simulink subsystem "TV_FLC"  (R2026a)
settings: Solver=VariableStepAuto
model mask{StrWheelRatio=Control.StrWheelRatio, Ku=Control.UndersteerGradient, L=Control.Wheelbase, rwheel=Control.WheelRad, Gr=Control.GearRatio, fis=Control.FuzzySystem, Kp=Control.KpMoment, tr=Control.RearTrack, alpha_max=Control.SlipTh, MotorT=Control.MotorTrq, MotorW=Control.MotorW, F=Control.F, Tmax=max(Control.MotorTrq)}
  mask prompts: StrWheelRatio "Steering Ratio"; Ku "Understeer Gradient"; L "WheelBase"; rwheel "Wheel Radius"; Gr "Gear ratio"; fis "Fuzzy Inference System"; Kp "Moment Coef"; tr "Rear Track"; alpha_max "Slip Threshold"; MotorT "Motor Map Torque"; MotorW "Motor Map RPM"; F "Moment to torque"; Tmax "Max Torque"
values from neighbouring files (symbols this model uses):
  Gr = 1/Vehicle.Powertrain.Driveline.Gearbox.ratio.Value    [sm_car_controlparam_FLCDYC.m]
  L = -Vehicle.Chassis.Body.sAxle2.Value(1)    [sm_car_controlparam_FLCDYC.m]
  rwheel = tire_param.DIMENSION.UNLOADED_RADIUS    [sm_car_controlparam_FLCDYC.m]
  tr = Vehicle.Chassis.Body.TrackRear.Value    [sm_car_controlparam_FLCDYC.m]
libraries: sl_discontinuities x7, simulink x1, fuzblock x1
settings Model: Creator=andrei  LastModifiedBy=andrei

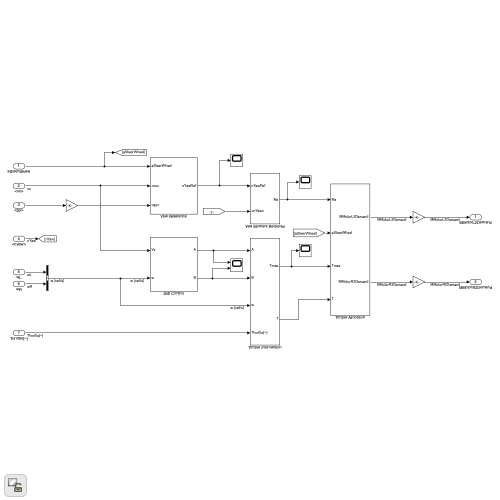
[thumbnail: Simulink's stored preview of the top-level diagram]
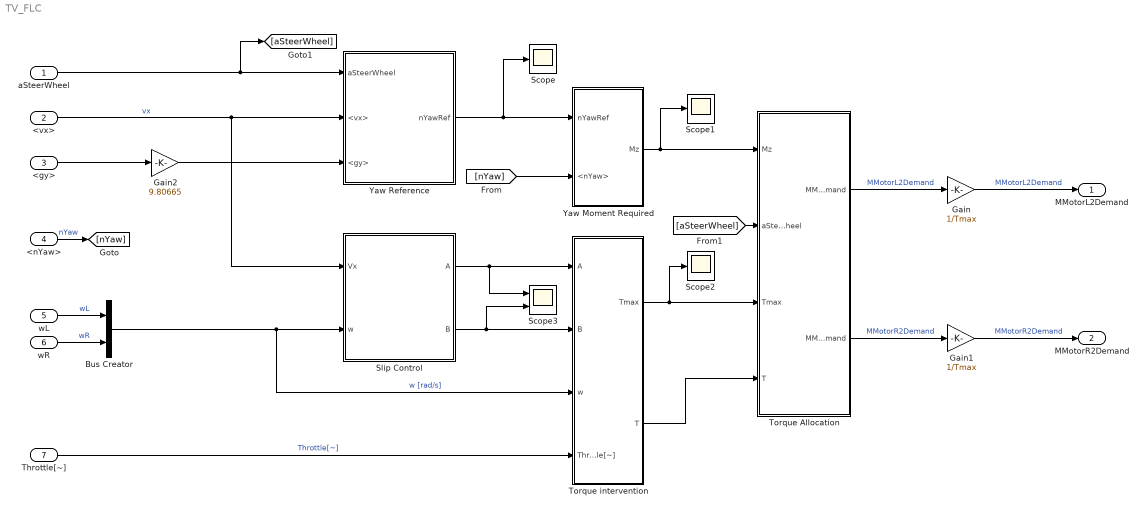
== system TV_FLC ==
  aSteerWheel : Inport  OutDataTypeStr=double  PortDimensions=1  SampleTime=0
  <vx> : Inport  Port=2  OutDataTypeStr=double  PortDimensions=1  SampleTime=0
  <gy> : Inport  Port=3  OutDataTypeStr=double  PortDimensions=1  SampleTime=0
  <nYaw> : Inport  Port=4  OutDataTypeStr=double  PortDimensions=1  SampleTime=0
  wL : Inport  Port=5  OutDataTypeStr=double  PortDimensions=1  SampleTime=0
  wR : Inport  Port=6  OutDataTypeStr=double  PortDimensions=1  SampleTime=0
  Throttle[~] : Inport  Port=7  OutDataTypeStr=double  PortDimensions=1  SampleTime=0
  Bus Creator : BusCreator  Inputs=2
  Gain : Gain  Gain=1/Tmax
  Gain1 : Gain  Gain=1/Tmax
  Gain2 : Gain  Gain=9.80665
  Scope : Scope
      settings: ActiveDisplayYMinimum=-0.70950113712266094  ActiveDisplayYMaximum=0.73291856494418972  DataLoggingVariableName=ScopeData12
  Scope1 : Scope
      settings: ActiveDisplayYMinimum=-1  ActiveDisplayYMaximum=1  DataLoggingVariableName=ScopeData13
  Scope2 : Scope
      settings: ActiveDisplayYMinimum=-1  ActiveDisplayYMaximum=1  DataLoggingVariableName=ScopeData3
  Scope3 : Scope  NumInputPorts=2
      settings: ActiveDisplayYMinimum=-0.025466589931511983  ActiveDisplayYMaximum=0.22919930938361235  DataLoggingVariableName=ScopeData9
  Slip Control : Subsystem
  Torque Allocation : Subsystem
  Torque intervention : Subsystem
  Yaw Moment Required : Subsystem
  Yaw Reference : Subsystem
  MMotorL2Demand : Outport  OutDataTypeStr=double  PortDimensions=1  SampleTime=0
  MMotorR2Demand : Outport  Port=2  OutDataTypeStr=double  PortDimensions=1  SampleTime=0
  wires:
  Torque Allocation/1(MMotorL2Demand) -> Gain/1  "MMotorL2Demand"
  <vx>/1 -> Yaw Reference/2(<vx>), Slip Control/1(Vx)  "vx"
  Slip Control/2(B) -> Torque intervention/2(B), Scope3/2
  <nYaw>/1 -> [nYaw]  "nYaw"
  Slip Control/1(A) -> Torque intervention/1(A), Scope3/1
  wL/1 -> Bus Creator/1  "wL"
  Yaw Moment Required/1(Mz) -> Torque Allocation/1(Mz), Scope1/1
  Throttle[~]/1 -> Torque intervention/4(Throttle[~])  "Throttle[~]"
  <gy>/1 -> Gain2/1
  Gain1/1 -> MMotorR2Demand/1  "MMotorR2Demand"
  [nYaw] -> Yaw Moment Required/2(<nYaw>)
  Bus Creator/1 -> Slip Control/2(w), Torque intervention/3(w)  "w [rad/s]"
  Gain/1 -> MMotorL2Demand/1  "MMotorL2Demand"
  Torque Allocation/2(MMotorR2Demand) -> Gain1/1  "MMotorR2Demand"
  Yaw Reference/1(nYawRef) -> Yaw Moment Required/1(nYawRef), Scope/1
  wR/1 -> Bus Creator/2  "wR"
  Torque intervention/1(Tmax) -> Torque Allocation/3(Tmax), Scope2/1
  Gain2/1 -> Yaw Reference/3(<gy>)
  Torque intervention/2(T) -> Torque Allocation/4(T)
  aSteerWheel/1 -> [aSteerWheel], Yaw Reference/1(aSteerWheel)
  [aSteerWheel] -> Torque Allocation/2(aSteerWheel)

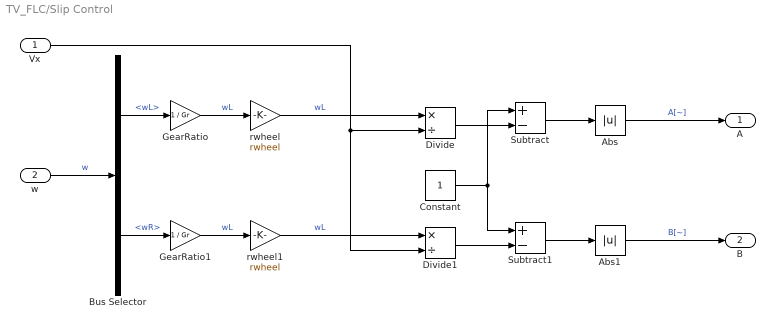
== system TV_FLC/Slip Control ==
  Vx : Inport
  w : Inport  Port=2
  Abs : Abs  SaturateOnIntegerOverflow=off
  Abs1 : Abs  SaturateOnIntegerOverflow=off
  Bus Selector : BusSelector  OutputSignals=wL,wR
  Constant : Constant
  Divide : Product  Inputs=*/
  Divide1 : Product  Inputs=*/
  GearRatio : Gain  Gain=1 / Gr
  GearRatio1 : Gain  Gain=1 / Gr
  Subtract : Sum  Inputs=+-
  Subtract1 : Sum  Inputs=+-
  rwheel : Gain  Gain=rwheel
  rwheel1 : Gain  Gain=rwheel
  A : Outport
  B : Outport  Port=2
  wires:
  GearRatio1/1 -> rwheel1/1  "wL"
  GearRatio/1 -> rwheel/1  "wL"
  rwheel1/1 -> Divide1/1  "wL"
  Bus Selector/1 -> GearRatio/1  "<wL>"
  w/1 -> Bus Selector/1  "w"
  Vx/1 -> Divide1/2, Divide/2
  Subtract/1 -> Abs/1
  Subtract1/1 -> Abs1/1
  rwheel/1 -> Divide/1  "wL"
  Bus Selector/2 -> GearRatio1/1  "<wR>"
  Constant/1 -> Subtract/1, Subtract1/1
  Divide/1 -> Subtract/2
  Divide1/1 -> Subtract1/2
  Abs/1 -> A/1  "A[~]"
  Abs1/1 -> B/1  "B[~]"

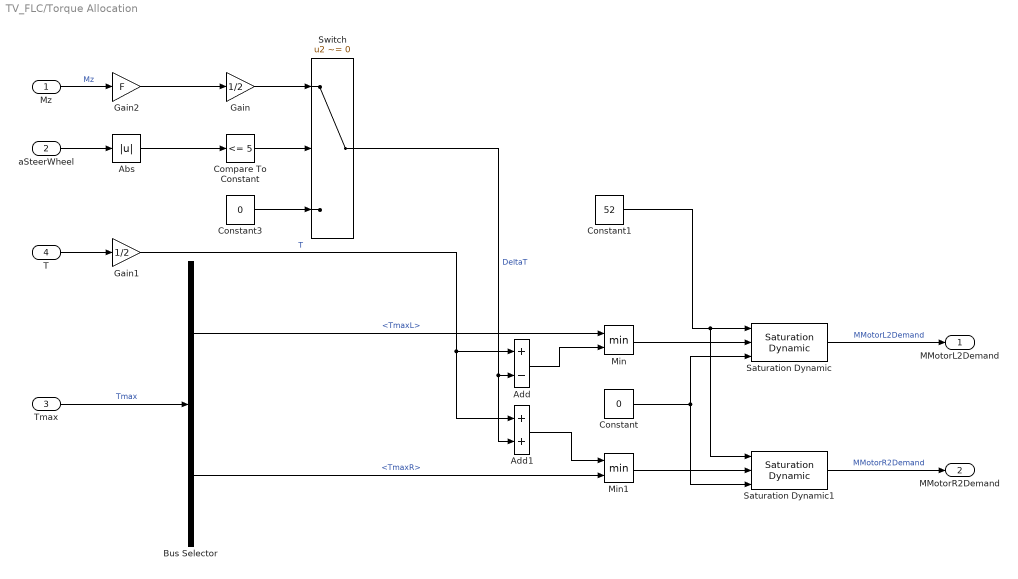
== system TV_FLC/Torque Allocation ==
  Mz : Inport
  aSteerWheel : Inport  Port=2
  Tmax : Inport  Port=3
  T : Inport  Port=4
  Abs : Abs  SaturateOnIntegerOverflow=off
  Add : Sum  Inputs=+-
  Add1 : Sum
  Bus Selector : BusSelector  OutputSignals=TmaxL,TmaxR
  Compare To Constant : simulink/Logic and Bit Operations/Compare To Constant  relop=<=  const=5  OutDataTypeStr=boolean
  Constant : Constant  Value=0
  Constant1 : Constant  Value=52
  Constant3 : Constant  Value=0
  Gain : Gain  Gain=1/2
  Gain1 : Gain  Gain=1/2
  Gain2 : Gain  Gain=F
  Min : MinMax  Inputs=2
  Min1 : MinMax  Inputs=2
  Saturation Dynamic : sl_discontinuities/Saturation Dynamic  OutMin=[]  OutMax=[]  OutDataTypeStr=Inherit: Same as second input  OutDataType=fixdt(1, 16)  OutScaling=2^-10  DoSatur=off
  Saturation Dynamic1 : sl_discontinuities/Saturation Dynamic  OutMin=[]  OutMax=[]  OutDataTypeStr=Inherit: Same as second input  OutDataType=fixdt(1, 16)  OutScaling=2^-10  DoSatur=off
  Switch : Switch  Criteria=u2 ~= 0  SaturateOnIntegerOverflow=off  InputSameDT=off
  MMotorL2Demand : Outport
  MMotorR2Demand : Outport  Port=2
  wires:
  Constant1/1 -> Saturation Dynamic/1, Saturation Dynamic1/1
  Gain2/1 -> Gain/1
  Min/1 -> Saturation Dynamic/2
  Min1/1 -> Saturation Dynamic1/2
  Gain/1 -> Switch/1
  Compare To Constant/1 -> Switch/2
  aSteerWheel/1 -> Abs/1
  Switch/1 -> Add/2, Add1/2  "DeltaT"
  Abs/1 -> Compare To Constant/1
  Constant3/1 -> Switch/3
  Constant/1 -> Saturation Dynamic1/3, Saturation Dynamic/3
  T/1 -> Gain1/1
  Mz/1 -> Gain2/1  "Mz"
  Gain1/1 -> Add/1, Add1/1  "T"
  Add1/1 -> Min1/1
  Add/1 -> Min/2
  Saturation Dynamic/1 -> MMotorL2Demand/1  "MMotorL2Demand"
  Saturation Dynamic1/1 -> MMotorR2Demand/1  "MMotorR2Demand"
  Tmax/1 -> Bus Selector/1  "Tmax"
  Bus Selector/1 -> Min/1  "<TmaxL>"
  Bus Selector/2 -> Min1/2  "<TmaxR>"

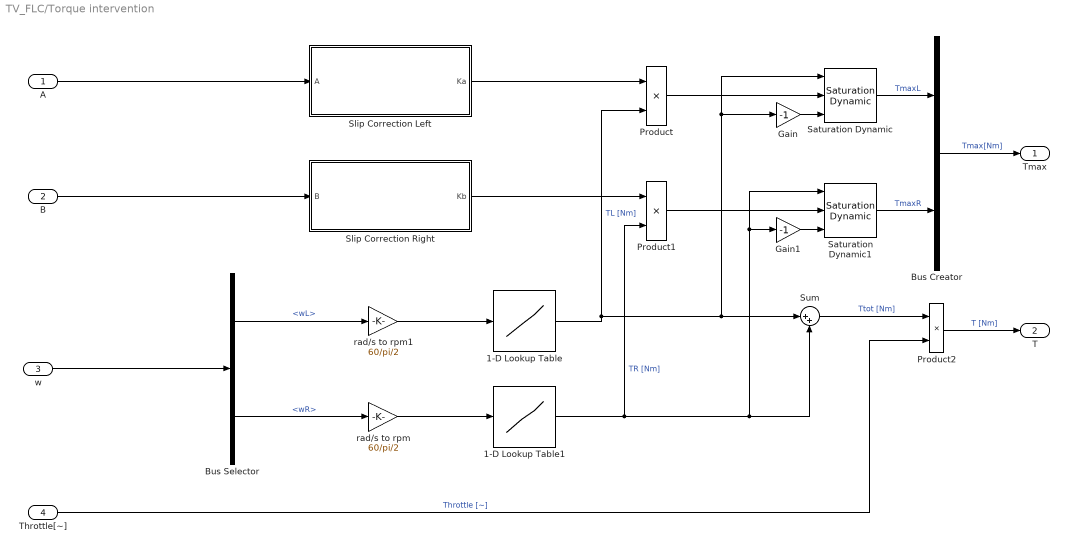
== system TV_FLC/Torque intervention ==
  A : Inport
  B : Inport  Port=2
  w : Inport  Port=3
  Throttle[~] : Inport  Port=4
  1-D Lookup Table : Lookup_n-D  NumberOfTableDimensions=1  BreakpointsForDimension1=MotorW  Table=MotorT  InternalRulePriority=Speed  RndMeth=Simplest
  1-D Lookup Table1 : Lookup_n-D  NumberOfTableDimensions=1  BreakpointsForDimension1=MotorW  Table=MotorT  InternalRulePriority=Speed  RndMeth=Simplest
  Bus Creator : BusCreator  Inputs=2
  Bus Selector : BusSelector  OutputSignals=wL,wR
  Gain : Gain  Gain=-1
  Gain1 : Gain  Gain=-1
  Product : Product
  Product1 : Product
  Product2 : Product
  Saturation Dynamic : sl_discontinuities/Saturation Dynamic  OutMin=[]  OutMax=[]  OutDataTypeStr=Inherit: Same as second input  OutDataType=fixdt(1, 16)  OutScaling=2^-10  DoSatur=off
  Saturation Dynamic1 : sl_discontinuities/Saturation Dynamic  OutMin=[]  OutMax=[]  OutDataTypeStr=Inherit: Same as second input  OutDataType=fixdt(1, 16)  OutScaling=2^-10  DoSatur=off
  Slip Correction Left : Subsystem
  Slip Correction Right : Subsystem
  Sum : Sum  Inputs=|++
  rad/s to rpm : Gain  Gain=60/pi/2
  rad/s to rpm1 : Gain  Gain=60/pi/2
  Tmax : Outport
  T : Outport  Port=2
  wires:
  Throttle[~]/1 -> Product2/2  "Throttle [~]"
  Sum/1 -> Product2/1  "Ttot [Nm]"
  Product2/1 -> T/1  "T [Nm]"
  A/1 -> Slip Correction Left/1(A)
  B/1 -> Slip Correction Right/1(B)
  Slip Correction Left/1(Ka) -> Product/1
  Slip Correction Right/1(Kb) -> Product1/1
  Product/1 -> Saturation Dynamic/2
  Gain/1 -> Saturation Dynamic/3
  Gain1/1 -> Saturation Dynamic1/3
  Product1/1 -> Saturation Dynamic1/2
  Saturation Dynamic/1 -> Bus Creator/1  "TmaxL"
  Saturation Dynamic1/1 -> Bus Creator/2  "TmaxR"
  Bus Creator/1 -> Tmax/1  "Tmax[Nm]"
  rad/s to rpm/1 -> 1-D Lookup Table1/1
  rad/s to rpm1/1 -> 1-D Lookup Table/1
  w/1 -> Bus Selector/1
  Bus Selector/1 -> rad/s to rpm1/1  "<wL>"
  Bus Selector/2 -> rad/s to rpm/1  "<wR>"
  1-D Lookup Table/1 -> Product/2, Saturation Dynamic/1, Gain/1, Sum/1  "TL [Nm]"
  1-D Lookup Table1/1 -> Product1/2, Gain1/1, Saturation Dynamic1/1, Sum/2  "TR [Nm]"

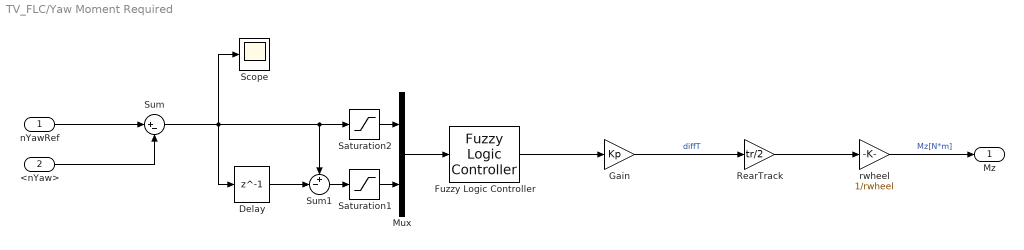
== system TV_FLC/Yaw Moment Required ==
  nYawRef : Inport
  <nYaw> : Inport  Port=2
  Delay : Delay  DelayLength=1  InputProcessing=Columns as channels (frame based)
  Fuzzy Logic Controller : fuzblock/Fuzzy Logic  Controller  FIS=fis  OutputSampleNumber=200  DataType=double  UseLookupTable=off  NumBreakpoints=10  FuzzifiedInputs=off  RuleFiringStrengths=off  RuleOutputs=off  AggregatedOutputs=off  SimulateUsing=Code generation  OutOfRangeInputValueMessage=warning  NoRuleFiredMessage=warning  EmptyOutputFuzzySetMessage=warning
  Gain : Gain  Gain=Kp
  Mux : Mux  Inputs=2
  RearTrack : Gain  Gain=tr/2
  Saturation1 : Saturate  UpperLimit=1  LowerLimit=-1
  Saturation2 : Saturate  UpperLimit=1  LowerLimit=-1
  Scope : Scope
      settings: ActiveDisplayYMinimum=-1  ActiveDisplayYMaximum=1  DataLoggingVariableName=ScopeData5
  Sum : Sum  Inputs=|+-
  Sum1 : Sum  Inputs=+-|
  rwheel : Gain  Gain=1/rwheel
  Mz : Outport
  wires:
  nYawRef/1 -> Sum/1
  <nYaw>/1 -> Sum/2
  Delay/1 -> Sum1/2
  Mux/1 -> Fuzzy Logic Controller/1
  Fuzzy Logic Controller/1 -> Gain/1
  rwheel/1 -> Mz/1  "Mz[N*m]"
  RearTrack/1 -> rwheel/1
  Sum/1 -> Saturation2/1, Sum1/1, Delay/1, Scope/1
  Saturation2/1 -> Mux/1
  Sum1/1 -> Saturation1/1
  Saturation1/1 -> Mux/2
  Gain/1 -> RearTrack/1  "diffT"

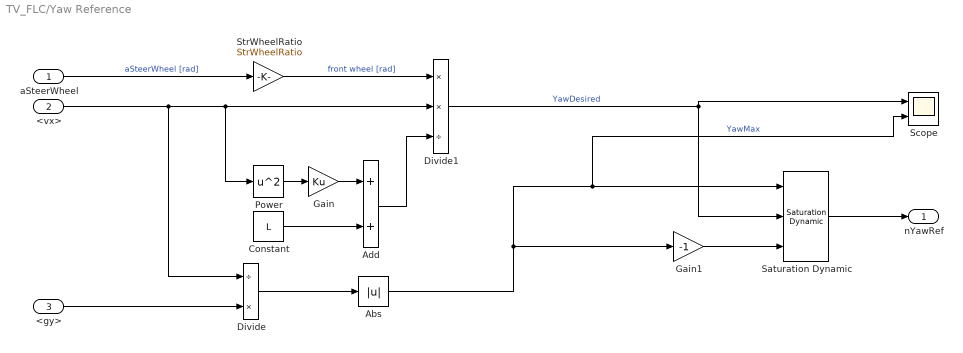
== system TV_FLC/Yaw Reference ==
  aSteerWheel : Inport
  <vx> : Inport  Port=2
  <gy> : Inport  Port=3
  Abs : Abs  SaturateOnIntegerOverflow=off
  Add : Sum
  Constant : Constant  Value=L
  Divide : Product  Inputs=/*
  Divide1 : Product  Inputs=**/
  Gain : Gain  Gain=Ku
  Gain1 : Gain  Gain=-1
  Power : Math  Operator=square
  Saturation Dynamic : sl_discontinuities/Saturation Dynamic  OutMin=[]  OutMax=[]  OutDataTypeStr=Inherit: Same as second input  OutDataType=fixdt(1, 16)  OutScaling=2^-10  DoSatur=off
  Scope : Scope  NumInputPorts=2
      settings: ActiveDisplayYMinimum=-0.77317443098288718  ActiveDisplayYMaximum=1.3059782096862267  DataLoggingVariableName=ScopeData4
  StrWheelRatio : Gain  Gain=StrWheelRatio
  nYawRef : Outport
  wires:
  aSteerWheel/1 -> StrWheelRatio/1  "aSteerWheel [rad]"
  StrWheelRatio/1 -> Divide1/1  "front wheel [rad]"
  <vx>/1 -> Divide1/2, Power/1, Divide/1
  <gy>/1 -> Divide/2
  Divide/1 -> Abs/1
  Saturation Dynamic/1 -> nYawRef/1
  Abs/1 -> Saturation Dynamic/1, Scope/2, Gain1/1  "YawMax"
  Gain1/1 -> Saturation Dynamic/3
  Divide1/1 -> Saturation Dynamic/2, Scope/1  "YawDesired"
  Power/1 -> Gain/1
  Gain/1 -> Add/1
  Constant/1 -> Add/2
  Add/1 -> Divide1/3

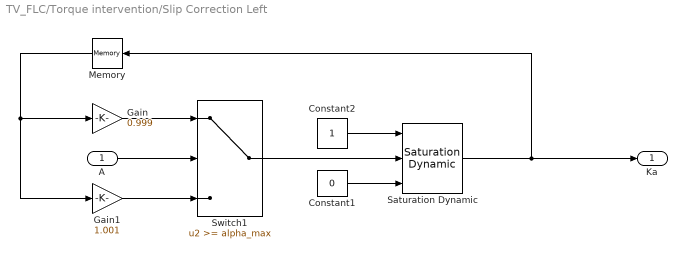
== system TV_FLC/Torque intervention/Slip Correction Left ==
  A : Inport
  Constant1 : Constant  Value=0
  Constant2 : Constant
  Gain : Gain  Gain=0.999
  Gain1 : Gain  Gain=1.001
  Memory : Memory  InitialCondition=1
  Saturation Dynamic : sl_discontinuities/Saturation Dynamic  OutMin=[]  OutMax=[]  OutDataTypeStr=Inherit: Same as second input  OutDataType=fixdt(1, 16)  OutScaling=2^-10  DoSatur=off
  Switch1 : Switch  Threshold=alpha_max  SaturateOnIntegerOverflow=off  InputSameDT=off
  Ka : Outport
  wires:
  Gain/1 -> Switch1/1
  Switch1/1 -> Saturation Dynamic/2
  Constant1/1 -> Saturation Dynamic/3
  Memory/1 -> Gain/1, Gain1/1
  Gain1/1 -> Switch1/3
  Saturation Dynamic/1 -> Ka/1, Memory/1
  A/1 -> Switch1/2
  Constant2/1 -> Saturation Dynamic/1

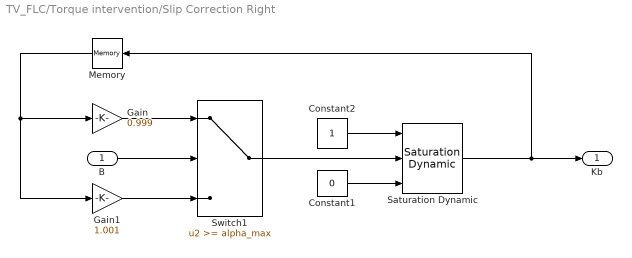
== system TV_FLC/Torque intervention/Slip Correction Right ==
  B : Inport
  Constant1 : Constant  Value=0
  Constant2 : Constant
  Gain : Gain  Gain=0.999
  Gain1 : Gain  Gain=1.001
  Memory : Memory  InitialCondition=1
  Saturation Dynamic : sl_discontinuities/Saturation Dynamic  OutMin=[]  OutMax=[]  OutDataTypeStr=Inherit: Same as second input  OutDataType=fixdt(1, 16)  OutScaling=2^-10  DoSatur=off
  Switch1 : Switch  Threshold=alpha_max  SaturateOnIntegerOverflow=off  InputSameDT=off
  Kb : Outport
  wires:
  Constant2/1 -> Saturation Dynamic/1
  B/1 -> Switch1/2
  Saturation Dynamic/1 -> Kb/1, Memory/1
  Gain1/1 -> Switch1/3
  Memory/1 -> Gain/1, Gain1/1
  Constant1/1 -> Saturation Dynamic/3
  Switch1/1 -> Saturation Dynamic/2
  Gain/1 -> Switch1/1
